simulink model "rfdc_V0_2"  (R2018a)
settings: Solver=VariableStepAuto  StartTime=0.0  StopTime=10.0  RelTol=1e-3
libraries: xbsIndex_r4 x4
settings Model: Creator=wei  LastModifiedBy=wei

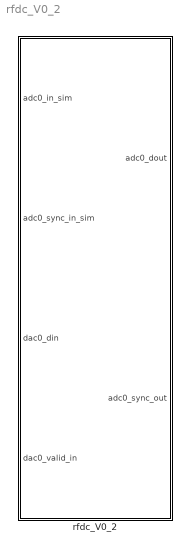
== system rfdc_V0_2 ==
  rfdc_V0_2 : Subsystem  Tag=xps:rfdc_V0_2  mask(rfdc){sys_config=1*1-ADC: R2R  DAC: R2R, adc_sample_rate=2048}
      mask prompts: sys_config "System Configuration"; adc_sample_rate "ADC Clock Rate(MHz)"
      mask help: This is for implementing RFDC core in RFSOC. The dac sample rate is double of the adc sample rate.
      mask init:
      | rfdc_v0_2_init(gcb,...
      |     'sys_config',sys_config,...
      |     'adc_sample_rate',adc_sample_rate);
      mask TypeOptions sys_config: 1*1-ADC: R2R  DAC: R2R | 2*2-ADC: R2R  DAC: R2R | 4*4-ADC: R2R  DAC: R2R | 8*8-ADC: R2R  DAC: R2R
      mask TypeOptions adc_sample_rate: 2048

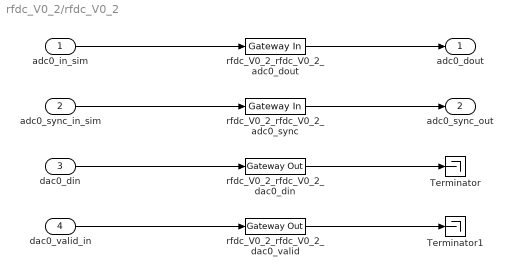
== system rfdc_V0_2/rfdc_V0_2 ==
  adc0_in_sim : Inport
  adc0_sync_in_sim : Inport  Port=2
  dac0_din : Inport  Port=3
  dac0_valid_in : Inport  Port=4
  Terminator : Terminator
  Terminator1 : Terminator
  rfdc_V0_2_rfdc_V0_2_adc0_dout : xbsIndex_r4/Gateway In  gui_display_data_type=Fixed-point  arith_type=Unsigned  n_bits=128  bin_pt=0  preci_type=Single  exp_width=8  frac_width=24  rows=1  columns=1  quantization=Truncate  overflow=Wrap  period=1  UseAsADC=off  ADCChannel='1'  interface=None  automatic_assignment=on  address_offset=hex2dec('00')  intf_name=''  intf_description=''  default_value=0  timing_constraint=None  locs_specified=off  LOCs={}  io_standard={}  inherit_from_input=off  hdl_port=on  dbl_ovrd=off  block_type=gatewayin
  rfdc_V0_2_rfdc_V0_2_adc0_sync : xbsIndex_r4/Gateway In  gui_display_data_type=Fixed-point  arith_type=Boolean  n_bits=1  bin_pt=0  preci_type=Single  exp_width=8  frac_width=24  rows=1  columns=1  quantization=Truncate  overflow=Wrap  period=1  UseAsADC=off  ADCChannel='1'  interface=None  automatic_assignment=on  address_offset=hex2dec('00')  intf_name=''  intf_description=''  default_value=0  timing_constraint=None  locs_specified=off  LOCs={}  io_standard={}  inherit_from_input=off  hdl_port=on  dbl_ovrd=off  block_type=gatewayin
  rfdc_V0_2_rfdc_V0_2_dac0_din : xbsIndex_r4/Gateway Out  inherit_from_input=off  hdl_port=on  rows=1  columns=1  UseAsDAC=off  DACChannel='1'  interface=None  automatic_assignment=on  address_offset=hex2dec('00')  intf_name=''  intf_description=''  timing_constraint=None  locs_specified=off  LOCs={}  io_standard={}  block_type=gatewayout
  rfdc_V0_2_rfdc_V0_2_dac0_valid : xbsIndex_r4/Gateway Out  inherit_from_input=off  hdl_port=on  rows=1  columns=1  UseAsDAC=off  DACChannel='1'  interface=None  automatic_assignment=on  address_offset=hex2dec('00')  intf_name=''  intf_description=''  timing_constraint=None  locs_specified=off  LOCs={}  io_standard={}  block_type=gatewayout
  adc0_dout : Outport
  adc0_sync_out : Outport  Port=2
  wires:
  adc0_in_sim/1 -> rfdc_V0_2_rfdc_V0_2_adc0_dout/1
  rfdc_V0_2_rfdc_V0_2_adc0_dout/1 -> adc0_dout/1
  adc0_sync_in_sim/1 -> rfdc_V0_2_rfdc_V0_2_adc0_sync/1
  rfdc_V0_2_rfdc_V0_2_adc0_sync/1 -> adc0_sync_out/1
  dac0_din/1 -> rfdc_V0_2_rfdc_V0_2_dac0_din/1
  rfdc_V0_2_rfdc_V0_2_dac0_din/1 -> Terminator/1
  dac0_valid_in/1 -> rfdc_V0_2_rfdc_V0_2_dac0_valid/1
  rfdc_V0_2_rfdc_V0_2_dac0_valid/1 -> Terminator1/1
